simulink model "Mockup_Calibration"  (R2018b)
settings: Solver=VariableStepAuto  StartTime=0.0  StopTime=10.0  RelTol=1e-3
libraries: simulink x2, dspstat3 x1, dspnetwork x1
settings Model: Creator=anton  LastModifiedBy=anton

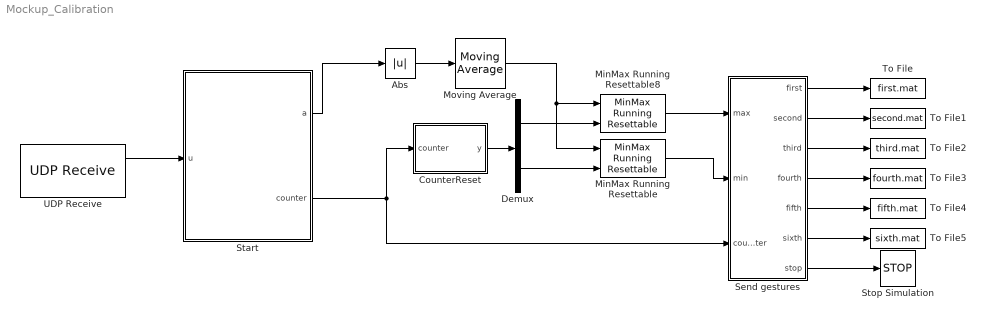
== system Mockup_Calibration ==
  Abs : Abs
  "CounterReset " : MATLAB Function  TreatAsAtomicUnit=on
  Demux : Demux  Outputs=2
  MinMax Running Resettable : simulink/Math Operations/MinMax Running Resettable  Function=min  vinit=1000
  MinMax Running Resettable8 : simulink/Math Operations/MinMax Running Resettable  Function=max  vinit=0
  Moving Average : dspstat3/Moving Average  Method=Sliding window  ForgettingFactorPort=off  SpecifyWindowLength=on  WindowLength=50  ForgettingFactor=0.9  SimulateUsing=Code generation
  "Send gestures " : MATLAB Function  TreatAsAtomicUnit=on
  "Start " : MATLAB Function  TreatAsAtomicUnit=on
  Stop Simulation : Stop
  To File : ToFile  Filename=first.mat  MatrixName=fist
  To File1 : ToFile  Filename=second.mat  MatrixName=fist
  To File2 : ToFile  Filename=third.mat  MatrixName=fist
  To File3 : ToFile  Filename=fourth.mat  MatrixName=fist
  To File4 : ToFile  Filename=fifth.mat  MatrixName=fist
  To File5 : ToFile  Filename=sixth.mat  MatrixName=fist
  UDP Receive : dspnetwork/UDP Receive  localURL='0.0.0.0'  localPort=54000  remoteURL='0.0.0.0'  remotePort=-1  recvBufferSize=128  dims=255  signalDatatype=int8  isVarSize=off  showBlockingTime=off  blockingTime=0  sampletime=0.02  blockPlatform=[]
      settings: SourceProductName=DSP System Toolbox  SourceProductBaseCode=DS
  wires:
  Moving Average/1 -> MinMax Running Resettable/1, MinMax Running Resettable8/1
  "Send gestures "/7(stop) -> Stop Simulation/1
  "Start "/1(a) -> Abs/1
  MinMax Running Resettable8/1 -> "Send gestures "/1(max)
  Abs/1 -> Moving Average/1
  "Start "/2(counter) -> "CounterReset "/1(counter), "Send gestures "/3(counter)
  UDP Receive/1 -> "Start "/1(u)
  MinMax Running Resettable/1 -> "Send gestures "/2(min)
  Demux/1 -> MinMax Running Resettable8/2
  "CounterReset "/1(y) -> Demux/1
  Demux/2 -> MinMax Running Resettable/2
  "Send gestures "/1(first) -> To File/1
  "Send gestures "/2(second) -> To File1/1
  "Send gestures "/3(third) -> To File2/1
  "Send gestures "/4(fourth) -> To File3/1
  "Send gestures "/5(fifth) -> To File4/1
  "Send gestures "/6(sixth) -> To File5/1

== matlab function Mockup_Calibration/Start  ==
  data: u input; a output; counter output
%a is the output of this block, and fcn(u) is the input required
function [a,counter]  = fcn(u)

persistent count 
if isempty(count)
   count =0; 
end

% We could error message in case we are receiving zero vector
if isempty(u)==0  
   count = count+1; 
end

counter=count;
%Below the output a is specified as the 3 row of the 8x1 input vector u
a = u(1,:);
b = u(2,:);
c = u(3,:);
d = u(4,:);
e = u(5,:);
f = u(6,:);
g = u(7,:);
h = u(8,:);

% a = u(1);
% b = u(2);
% c = u(3);
% d = u(4);
% e = u(5);
% f = u(6);
% g = u(7);
% h = u(8);

== matlab function Mockup_Calibration/Send gestures  ==
  data: max input; min input; first output; counter input; second output; third output; fourth output; fifth output; sixth output; stop output
function [first,second,third,fourth,fifth,sixth,stop] = fcn(max, min, counter)
    
    stop=0;
    first=zeros(1,16);
    second=zeros(1,16);
    third=zeros(1,16);
    fourth=zeros(1,16);
    fifth=zeros(1,16);
    sixth=zeros(1,16);

if counter==250
    first=[maxA minA maxB minB maxC minC maxD minD maxE minE maxF minF maxG minG maxH minH];

elseif counter==750
    second=[maxA minA maxB minB maxC minC maxD minD maxE minE maxF minF maxG minG maxH minH];

elseif counter==1250
    third=[maxA minA maxB minB maxC minC maxD minD maxE minE maxF minF maxG minG maxH minH];

elseif counter==1750
    fourth=[maxA minA maxB minB maxC minC maxD minD maxE minE maxF minF maxG minG maxH minH];
    
elseif counter==2250
    fifth=[maxA minA maxB minB maxC minC maxD minD maxE minE maxF minF maxG minG maxH minH];
    
elseif counter==2750
    sixth=[maxA minA maxB minB maxC minC maxD minD maxE minE maxF minF maxG minG maxH minH];
    pause(0.5);
    stop=1;
     
end

== matlab function Mockup_Calibration/CounterReset  ==
  data: counter input; y output
function y = fcn(counter)
if counter==50
    y=[1 1 1 1 1 1 1 1 1 1 1 1 1 1 1 1];
elseif counter==550
    y=[1 1 1 1 1 1 1 1 1 1 1 1 1 1 1 1];
elseif counter==1050
    y=[1 1 1 1 1 1 1 1 1 1 1 1 1 1 1 1];
elseif counter==1550
    y=[1 1 1 1 1 1 1 1 1 1 1 1 1 1 1 1];
elseif counter==2050
    y=[1 1 1 1 1 1 1 1 1 1 1 1 1 1 1 1];
elseif counter==2550
    y=[1 1 1 1 1 1 1 1 1 1 1 1 1 1 1 1];

    
else 
    y=zeros(1,16)
end
